simulink model "DC_motor_params_mf"  (R2023b)
settings: Solver=ode4  StartTime=0.0  StopTime=10  FixedStep=0.0005  RelTol=1e-3
values from neighbouring files (symbols this model uses):
  B = 0.0003    [DC_motor_params.m]    (also in LPF_ex.m)
  J = 2.09*10^(-5)    (= 2.09e-05)    [DC_motor_params.m]    (also in LPF_ex.m)
  Kb = 0.042    [DC_motor_params.m]    (also in LPF_ex.m)
  Kt = 0.042    [DC_motor_params.m]    (also in LPF_ex.m)
  L = 1.16    [DC_motor_params.m]    (also in LPF_ex.m)
  R = 8.4    [DC_motor_params.m]    (also in LPF_ex.m)
settings Model: Creator=SJ  LastModifiedBy=SJ

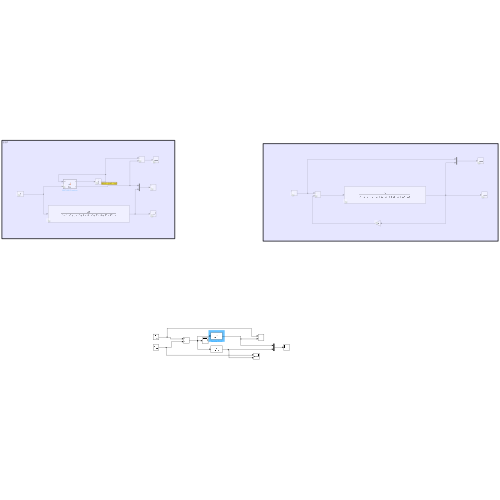
[thumbnail: Simulink's stored preview of the top-level diagram]
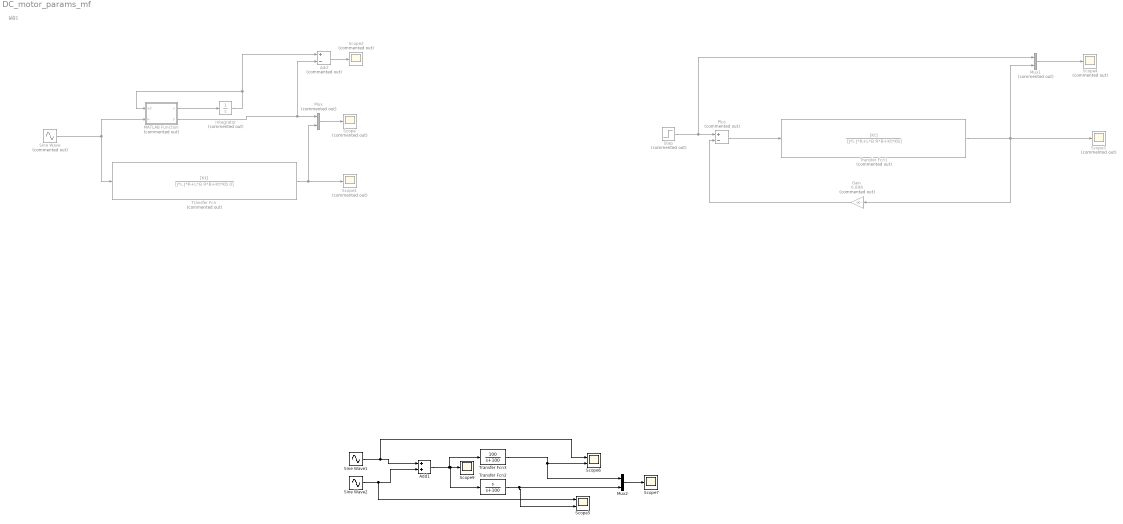
== system DC_motor_params_mf ==
  note: 실습1
  Add : Sum  Commented=on  Inputs=+-
  Add1 : Sum
  Gain : Gain  Commented=on  Gain=0.898
  Integrator : Integrator  Commented=on
  MATLAB Function : MATLAB Function  Commented=on  TreatAsAtomicUnit=on
  Mux : Mux  Commented=on  Inputs=2
  Mux1 : Mux  Commented=on  Inputs=2
  Mux2 : Mux  Inputs=2
  Plus : Sum  Commented=on  Inputs=+-
  Scope{,1..4} (5 alike) : Scope  Commented=on
  Scope5 : Scope  NumInputPorts=2
  Scope6 : Scope  NumInputPorts=2
  Scope7 : Scope
  Scope9 : Scope
  Sine Wave : Sin  Commented=on  SampleTime=0
  Sine Wave1 : Sin  SampleTime=0
  Sine Wave2 : Sin  Frequency=1000  SampleTime=0
  Step : Step  Commented=on  After=2  SampleTime=0
  Transfer Fcn : TransferFcn  Commented=on  Numerator=[Kt]  Denominator=[J*L J*R+L*B R*B+Kt*Kb 0]
  Transfer Fcn1 : TransferFcn  Commented=on  Numerator=[Kt]  Denominator=[J*L J*R+L*B R*B+Kt*Kb]
  Transfer Fcn2 : TransferFcn  Numerator=[1 0]  Denominator=[1 100]
  Transfer Fcn3 : TransferFcn  Numerator=[100]  Denominator=[1 100]
  wires:
  Sine Wave/1 -> MATLAB Function/2(u), Transfer Fcn/1
  MATLAB Function/1(x) -> Integrator/1
  Integrator/1 -> Add/1, MATLAB Function/1(xd)
  Transfer Fcn/1 -> Mux/2, Scope1/1
  MATLAB Function/2(y) -> Add/2, Mux/1
  Mux/1 -> Scope/1
  Add/1 -> Scope2/1
  Step/1 -> Mux1/1, Plus/1
  Plus/1 -> Transfer Fcn1/1
  Transfer Fcn1/1 -> Gain/1, Mux1/2, Scope3/1
  Mux1/1 -> Scope4/1
  Gain/1 -> Plus/2
  Sine Wave1/1 -> Scope6/1, Add1/1
  Sine Wave2/1 -> Scope5/1, Add1/2
  Add1/1 -> Scope9/1, Transfer Fcn2/1, Transfer Fcn3/1
  Transfer Fcn3/1 -> Mux2/1, Scope6/2
  Transfer Fcn2/1 -> Scope5/2, Mux2/2
  Mux2/1 -> Scope7/1

== matlab function DC_motor_params_mf/MATLAB Function ==
  data: xd input size=3; x output; u input; y output
function [x,y] = fcn(xd, u)

J=2.09*10^(-5);
Kb=0.042;
Kt=0.042;
R=8.4;
L=1.16;
B=0.0003;
%xd는 동역학의 상태 p13
x = [xd(2);
    Kt/J*xd(3)-B/J*xd(2);
    -R/L*xd(3)-Kb/L*xd(2)+1/L*u];
y = xd(1);
